simulink model "controlSystem"  (R2024b)
settings: Solver=VariableStepAuto  StartTime=0.0  StopTime=50  RelTol=1e-3
values from neighbouring files (symbols this model uses):
  H = 1 ./ sqrt(1 + (f_plot ./ fc).^2)    [SensorNoiseDetection.m]    (also in modeling.m = tf(num, den) * K)
  Kd = 3.99642371709311    (= 3.99642371709)    [modeling.m]
  Ki = 1.10967723382933    (= 1.10967723383)    [modeling.m]
  Kp = 5.27508301369566    (= 5.2750830137)    [modeling.m]
settings Model: Creator=bolinsfe  LastModifiedBy=bolinsfe

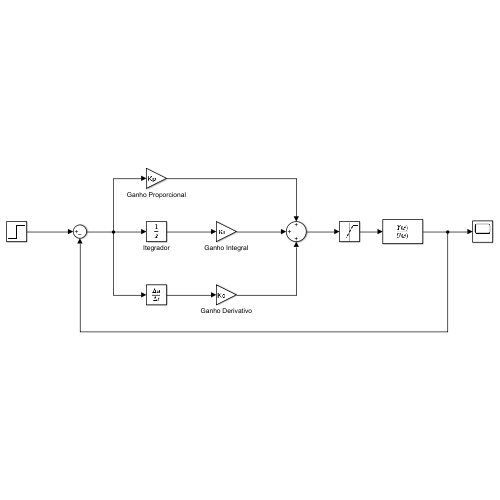
[thumbnail: Simulink's stored preview of the top-level diagram]
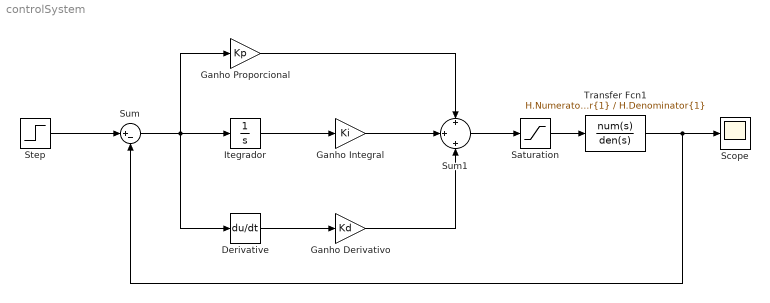
== system controlSystem ==
  Derivative : Derivative
  Ganho Derivativo : Gain  Gain=Kd
  Ganho Integral : Gain  Gain=Ki
  Ganho Proporcional : Gain  Gain=Kp
  Itegrador : Integrator
  Saturation : Saturate  UpperLimit=30  LowerLimit=-30
  Scope : Scope
  Step : Step  Time=0.010  SampleTime=0
  Sum : Sum  Inputs=|+-
  Sum1 : Sum  Inputs=+|+|+
  Transfer Fcn1 : TransferFcn  Numerator=H.Numerator{1}  Denominator=H.Denominator{1}
  wires:
  Step/1 -> Sum/1
  Sum/1 -> Derivative/1, Itegrador/1, Ganho Proporcional/1
  Ganho Proporcional/1 -> Sum1/1
  Saturation/1 -> Transfer Fcn1/1
  Sum1/1 -> Saturation/1
  Transfer Fcn1/1 -> Scope/1, Sum/2
  Itegrador/1 -> Ganho Integral/1
  Ganho Integral/1 -> Sum1/2
  Derivative/1 -> Ganho Derivativo/1
  Ganho Derivativo/1 -> Sum1/3
